simulink subsystem "OrientationAndMotorsSubsystem"  (R2023b)
settings: Solver=VariableStepAuto  StartTime=0.0  StopTime=10.0  RelTol=1e-3
values from neighbouring files (symbols this model uses):
  b = 192.3208*10^(-7)    (= 1.923208e-05)    [drone_input_params.m]
  d = 4.003*10^(-7)    (= 4.003e-07)    [drone_input_params.m]
settings Model: Creator=FRESH  LastModifiedBy=FRESH

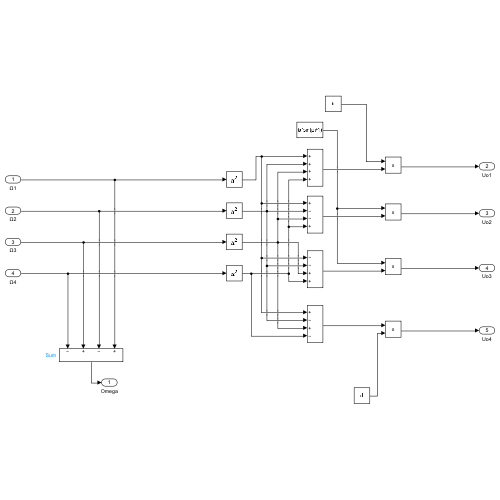
[thumbnail: Simulink's stored preview of the top-level diagram]
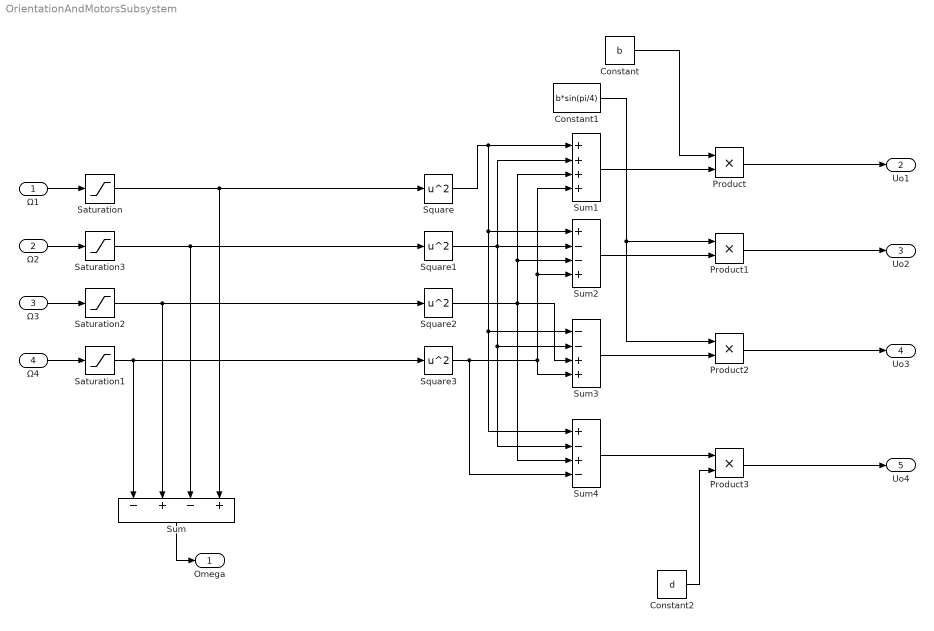
== system OrientationAndMotorsSubsystem ==
  Ω1 : Inport
  Ω2 : Inport  Port=2
  Ω3 : Inport  Port=3
  Ω4 : Inport  Port=4
  Constant : Constant  Value=b
  Constant1 : Constant  Value=b*sin(pi/4)
  Constant2 : Constant  Value=d
  Product{,1..3} (4 alike) : Product
  Saturation{,1..3} (4 alike) : Saturate  UpperLimit=inf  LowerLimit=0
  Square{,1..3} (4 alike) : Math  Operator=square
  Sum : Sum  Inputs=-+-+
  Sum1 : Sum  Inputs=++++
  Sum2 : Sum  Inputs=+--+
  Sum3 : Sum  Inputs=--++
  Sum4 : Sum  Inputs=+-+-
  Omega : Outport
  Uo1 : Outport  Port=2
  Uo2 : Outport  Port=3
  Uo3 : Outport  Port=4
  Uo4 : Outport  Port=5
  wires:
  Ω1/1 -> Saturation/1
  Ω2/1 -> Saturation3/1
  Ω3/1 -> Saturation2/1
  Ω4/1 -> Saturation1/1
  Sum/1 -> Omega/1
  Square/1 -> Sum4/1, Sum3/1, Sum2/1, Sum1/1
  Square1/1 -> Sum4/2, Sum3/2, Sum2/2, Sum1/2
  Square2/1 -> Sum4/3, Sum3/3, Sum2/3, Sum1/3
  Square3/1 -> Sum4/4, Sum3/4, Sum2/4, Sum1/4
  Constant/1 -> Product/1
  Sum1/1 -> Product/2
  Constant1/1 -> Product2/1, Product1/1
  Sum2/1 -> Product1/2
  Sum3/1 -> Product2/2
  Sum4/1 -> Product3/1
  Constant2/1 -> Product3/2
  Product/1 -> Uo1/1
  Product1/1 -> Uo2/1
  Product2/1 -> Uo3/1
  Product3/1 -> Uo4/1
  Saturation/1 -> Square/1, Sum/4
  Saturation3/1 -> Square1/1, Sum/3
  Saturation2/1 -> Square2/1, Sum/2
  Saturation1/1 -> Sum/1, Square3/1
